simulink model "SIMULINKA"  (R2023b)
settings: Solver=VariableStepAuto  StartTime=0.0  StopTime=1000  FixedStep=0.001  RelTol=1e-3
values from neighbouring files (symbols this model uses):
  h0 = h_vec(i)    [Bodes.m]    (also in TP1.m = 0.45)
  u0 = u_vec(i)    [Bodes.m]    (also in TP1.m = Qi/(a_salida*sqrt(2*g*h0)))
settings Model: Creator=aghersin  LastModifiedBy=tomig
settings SolverCC: AlgebraicLoopSolver=TrustRegion
settings DataIOCC: ReturnWorkspaceOutputs=off
settings OptimizationCC: LifeSpan=inf
settings DebuggingCC: UnconnectedInputMsg=warning  UnconnectedOutputMsg=warning  UnconnectedLineMsg=warning  SFExecutionAtInitializationDiag=none  ArithmeticOperatorsInVariantConditions=warning
settings ModelReferenceCC: EnableRefExpFcnMdlSchedulingChecks=on
settings SFSimCC: SimUseLocalCustomCode=off  CustomCodeUndefinedFunction=UseInterfaceOnly
settings RTWCC: RTWUseLocalCustomCode=off  DLArmComputeVersion=19.05
settings CodeAppCC: StateflowObjectComments=on

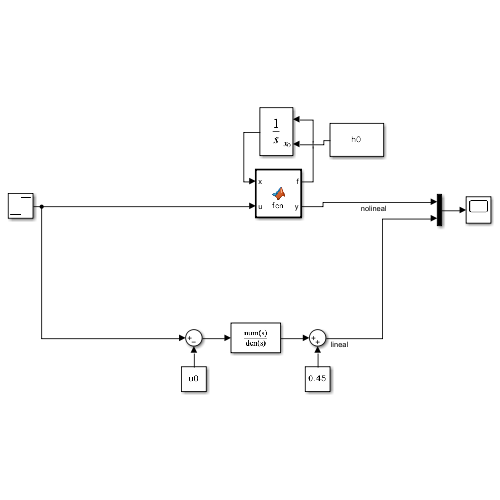
[thumbnail: Simulink's stored preview of the top-level diagram]
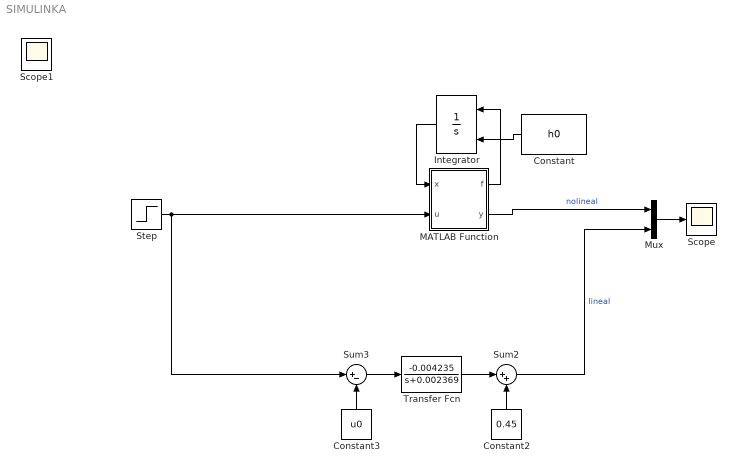
== system SIMULINKA ==
  Constant : Constant  Value=h0
  Constant2 : Constant  Value=0.45
  Constant3 : Constant  Value=u0
  Integrator : Integrator  InitialConditionSource=external
  MATLAB Function : MATLAB Function  TreatAsAtomicUnit=on
  Mux : Mux  Inputs=2
  Scope : Scope
  Step : Step  Before=u0  After=1.1*u0  SampleTime=0
  Sum2 : Sum  Inputs=|++
  Sum3 : Sum  Inputs=|+-
  Transfer Fcn : TransferFcn  Numerator=[-0.004235]  Denominator=[1 0.002369]
  Scope1 : Scope
  wires:
  Integrator/1 -> MATLAB Function/1(x)
  MATLAB Function/1(f) -> Integrator/1
  Constant/1 -> Integrator/2
  MATLAB Function/2(y) -> Mux/1  "nolineal"
  Transfer Fcn/1 -> Sum2/1
  Constant2/1 -> Sum2/2
  Sum3/1 -> Transfer Fcn/1
  Constant3/1 -> Sum3/2
  Sum2/1 -> Mux/2  "lineal"
  Step/1 -> MATLAB Function/2(u), Sum3/1
  Mux/1 -> Scope/1

== matlab function SIMULINKA/MATLAB Function ==
  data: x input; u input; f output; y output
function [f, y] = fcn(x, u)
    % Definición de constantes
    Qi = 8 * 0.001 / 60;  % Caudal constante de entrada (m^3/s)
    diam = 10.65 * 0.001; % Diámetro de la cañería de salida (m)
    l_chico = 0.1;        % Lado pequeño del tanque (m)
    l_grande = 0.4;       % Lado grande del tanque (m)
    h_tanque = 0.9;       % Altura del tanque (m)
    a_salida = pi * (diam / 2)^2; % Área de salida (m^2)
    g = 9.81;             % Gravedad (m/s^2)

    % Ecuación del sistema
    f = (Qi - (u * a_salida * sqrt(2 * g * x))) / ...
        ((l_chico)^2 + ((2 * l_chico * (l_grande - l_chico) * x) / h_tanque) + ...
        (((l_grande - l_chico) / h_tanque) * x)^2);
    
    % Salida del sistema
    y = x;
end
